simulink model "Pacejka_Tire_Model"  (R2018a)
settings: Solver=VariableStepAuto  StartTime=0.0  StopTime=10  RelTol=1e-3  EnableMultiTasking=on
undefined symbols (not defined in the file): sigbuilder_block
settings Model: Creator=oncel  LastModifiedBy=Dusseldo
settings DataIOCC: LimitDataPoints=on
settings OptimizationCC: LifeSpan=inf
settings DebuggingCC: AllowSymbolicDim=off  SFUnexpectedBacktrackingDiag=warning  SFNoUnconditionalDefaultTransitionDiag=warning  SFExecutionAtInitializationDiag=none
settings ModelReferenceCC: PropagateSignalLabelsOutOfModel=off
settings CodeAppCC: StateflowObjectComments=on
settings GRTTargetCC: TargetLangStandard=C89/C90 (ANSI)
settings ConfigComp: CovMetricSettings=dw  CovHtmlReporting=on  CovSaveCumulativeToWorkspaceVar=on  CovSaveSingleToWorkspaceVar=on  CovExternalEMLEnable=off

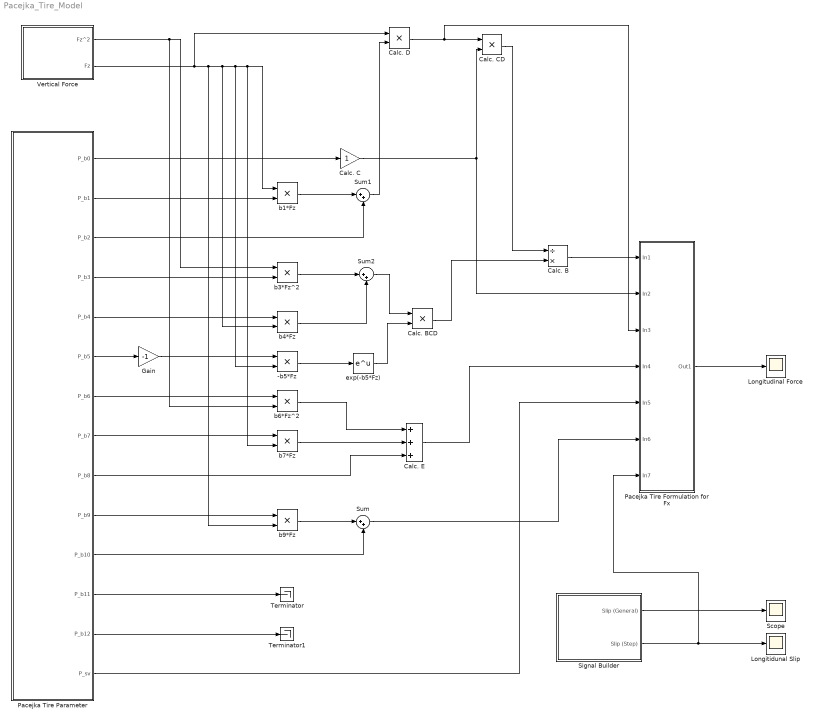
== system Pacejka_Tire_Model ==
  -b5*Fz : Product
  Calc. B : Product  Inputs=/*
  Calc. BCD : Product
  Calc. C : Gain
  Calc. CD : Product
  Calc. D : Product
  Calc. E : Sum  Inputs=+++
  Gain : Gain  Gain=-1
  Longitidunal Slip : Scope
  Longitudinal Force : Scope
  "Pacejka Tire Formulation for Fx " : Subsystem
  Pacejka Tire Parameter : Subsystem
  Scope : Scope
  Signal Builder : Subsystem  Tag=STV Subsys  LoadFcn=sigbuilder_block('load');  StartFcn=sigbuilder_block('start');  StopFcn=sigbuilder_block('stop');  ClipboardFcn=sigbuilder_block('clipboard');  mask(Sigbuilder block){tuvar=[0:10]}
      mask help: Simulink:masks:SigbuilderBlock_MD
      mask init:
      | if ~strcmp(get_param(bdroot(gcbh),'SimulationStatus'),'stopped') tuvar = sigbuilder_block('maskInit'); end
      settings: CopyFcn=sigbuilder_block('copy');  DeleteFcn=sigbuilder_block('delete');  ModelCloseFcn=sigbuilder_block('modelClose');  PreSaveFcn=sigbuilder_block('preSave');  PauseFcn=sigbuilder_block('pause');  ContinueFcn=sigbuilder_block('continue');  NameChangeFcn=sigbuilder_block('namechange');  OpenFcn=sigbuilder_block('open',[147.75 147.75 707.25 460.5 ]);  CloseFcn=sigbuilder_block('close');
      mask Display: plot(0, 0, 100, 100,[2, 2, 32, 32, 2], [68, 8, 8, 68, 68],[32, 2], [38, 38], [32, 19, 2],[53, 60, 44], [32, 17, 17, 2],[16, 16, 31, 31]);txt = getActiveGroup(gcbh);text(2, 100, txt,'verticalAlignment', 'top');
  Sum : Sum  Inputs=|++
  Sum1 : Sum  Inputs=|++
  Sum2 : Sum  Inputs=|++
  Terminator : Terminator
  Terminator1 : Terminator
  Vertical Force : Subsystem
  b1*Fz : Product
  b3*Fz^2 : Product
  b4*Fz : Product
  b6*Fz^2 : Product
  b7*Fz : Product
  b9*Fz : Product
  exp(-b5*Fz) : Math  SaturateOnIntegerOverflow=on
  wires:
  "Pacejka Tire Formulation for Fx "/1(Out1) -> Longitudinal Force/1
  Pacejka Tire Parameter/13(P_b12) -> Terminator1/1
  Pacejka Tire Parameter/12(P_b11) -> Terminator/1
  Pacejka Tire Parameter/1(P_b0) -> Calc. C/1
  Calc. C/1 -> "Pacejka Tire Formulation for Fx "/2(In2), Calc. CD/2
  Pacejka Tire Parameter/2("P_b1 ") -> b1*Fz/2
  Pacejka Tire Parameter/3(P_b2) -> Sum1/2
  b1*Fz/1 -> Sum1/1
  Sum1/1 -> Calc. D/2
  Pacejka Tire Parameter/4("P_b3 ") -> b3*Fz^2/2
  Vertical Force/1(Fz^2) -> b3*Fz^2/1, b6*Fz^2/2
  b3*Fz^2/1 -> Sum2/1
  Sum2/1 -> Calc. BCD/1
  Pacejka Tire Parameter/5(P_b4) -> b4*Fz/1
  Pacejka Tire Parameter/6(P_b5) -> Gain/1
  Gain/1 -> -b5*Fz/1
  Pacejka Tire Parameter/7(P_b6) -> b6*Fz^2/1
  Pacejka Tire Parameter/8(P_b7) -> b7*Fz/1
  b6*Fz^2/1 -> Calc. E/1
  Pacejka Tire Parameter/10(P_b9) -> b9*Fz/1
  Vertical Force/2(Fz) -> Calc. D/1, b9*Fz/2, -b5*Fz/2, b7*Fz/2, b1*Fz/1, b4*Fz/2
  b9*Fz/1 -> Sum/1
  Pacejka Tire Parameter/11(P_b10) -> Sum/2
  b7*Fz/1 -> Calc. E/2
  Pacejka Tire Parameter/9(P_b8) -> Calc. E/3
  b4*Fz/1 -> Sum2/2
  -b5*Fz/1 -> exp(-b5*Fz)/1
  exp(-b5*Fz)/1 -> Calc. BCD/2
  Calc. BCD/1 -> Calc. B/2
  Calc. CD/1 -> Calc. B/1
  Calc. B/1 -> "Pacejka Tire Formulation for Fx "/1(In1)
  Sum/1 -> "Pacejka Tire Formulation for Fx "/6(In6)
  Calc. E/1 -> "Pacejka Tire Formulation for Fx "/4(In4)
  Calc. D/1 -> "Pacejka Tire Formulation for Fx "/3(In3), Calc. CD/1
  Pacejka Tire Parameter/14(P_sv) -> "Pacejka Tire Formulation for Fx "/5(In5)
  Signal Builder/2(Slip (Step)) -> Longitidunal Slip/1, "Pacejka Tire Formulation for Fx "/7(In7)
  Signal Builder/1(Slip (General)) -> Scope/1

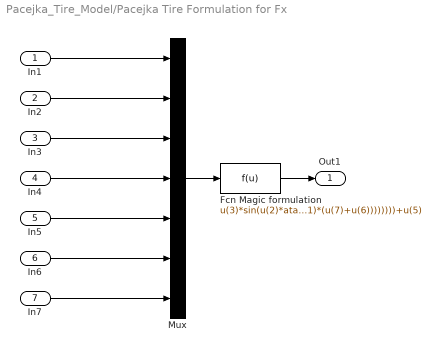
== system Pacejka_Tire_Model/Pacejka Tire Formulation for Fx  ==
  In1 : Inport
  In2 : Inport  Port=2
  In3 : Inport  Port=3
  In4 : Inport  Port=4
  In5 : Inport  Port=5
  In6 : Inport  Port=6
  In7 : Inport  Port=7
  Fcn Magic formulation : Fcn  Expr=u(3)*sin(u(2)*atan(u(1)*(u(7)+u(6)-u(4)*(u(1)*(u(7)+u(6)-atan(u(1)*(u(7)+u(6))))))))+u(5)
  Mux : Mux  Inputs=7
  Out1 : Outport
  wires:
  In1/1 -> Mux/1
  In2/1 -> Mux/2
  In3/1 -> Mux/3
  In4/1 -> Mux/4
  In5/1 -> Mux/5
  In6/1 -> Mux/6
  In7/1 -> Mux/7
  Mux/1 -> Fcn Magic formulation/1
  Fcn Magic formulation/1 -> Out1/1

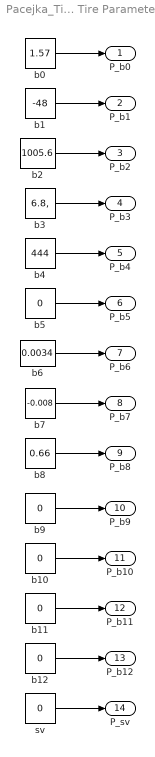
== system Pacejka_Tire_Model/Pacejka Tire Parameter ==
  b0 : Constant  Value=1.57
  b1 : Constant  Value=-48
  b{5,9..12} (5 alike) : Constant  Value=0
  b2 : Constant  Value=1005.6
  b3 : Constant  Value=6.8,
  b4 : Constant  Value=444
  b6 : Constant  Value=0.0034
  b7 : Constant  Value=-0.008
  b8 : Constant  Value=0.66
  sv : Constant  Value=0
  P_b0 : Outport
  "P_b1 " : Outport  Port=2
  P_b2 : Outport  Port=3
  "P_b3 " : Outport  Port=4
  P_b4 : Outport  Port=5
  P_b5 : Outport  Port=6
  P_b6 : Outport  Port=7
  P_b7 : Outport  Port=8
  P_b8 : Outport  Port=9
  P_b9 : Outport  Port=10
  P_b10 : Outport  Port=11
  P_b11 : Outport  Port=12
  P_b12 : Outport  Port=13
  P_sv : Outport  Port=14
  wires:
  b0/1 -> P_b0/1
  b1/1 -> "P_b1 "/1
  b2/1 -> P_b2/1
  b3/1 -> "P_b3 "/1
  b4/1 -> P_b4/1
  b5/1 -> P_b5/1
  b6/1 -> P_b6/1
  b7/1 -> P_b7/1
  b8/1 -> P_b8/1
  b9/1 -> P_b9/1
  b10/1 -> P_b10/1
  b11/1 -> P_b11/1
  b12/1 -> P_b12/1
  sv/1 -> P_sv/1

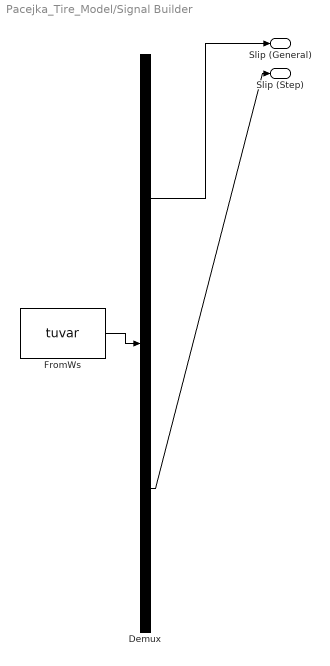
== system Pacejka_Tire_Model/Signal Builder ==
  Demux : Demux  Tag=STV Demux  Outputs=2
  FromWs : FromWorkspace  Tag=STV FromWs  VariableName=tuvar  SampleTime=0
      SigBuilderData=|
      | common.afterFinalStr = 'Extrapolate'
      | common.sampleTime = 0
      | dataSet.timeRange = [0 1]
      | dataSet.name = 'Slip'
      | sbobj.Groups.Name = 'Slip'
      | sbobj.Groups.Signals(1).Name = 'Slip (General)'
      | sbobj.Groups.Signals(1).XData = [0 1]
      | sbobj.Groups.Signals(1).YData = [-20 20]
      | sbobj.Groups.Signals(2).Name = 'Slip (Step)'
      | sbobj.Groups.Signals(2).XData = [0 0.2 0.8 1]
      | sbobj.Groups.Signals(2).YData = [-0.2 0.02 20 20]
      | sbobj.Groups.TimeRange = [0 1]
  Slip (General) : Outport  Tag=STV Outport
  Slip (Step) : Outport  Tag=STV Outport  Port=2
  wires:
  Demux/1 -> Slip (General)/1
  FromWs/1 -> Demux/1
  Demux/2 -> Slip (Step)/1

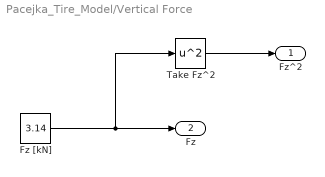
== system Pacejka_Tire_Model/Vertical Force ==
  Fz [kN] : Constant  Value=3.14
  Take Fz^2 : Math  Operator=square  SaturateOnIntegerOverflow=on
  Fz^2 : Outport
  Fz : Outport  Port=2
  wires:
  Fz [kN]/1 -> Take Fz^2/1, Fz/1
  Take Fz^2/1 -> Fz^2/1
